simulink model "GLR_recorded_data"  (R2024b)
settings: Solver=VariableStepAuto  StartTime=0.0  StopTime=45  RelTol=1e-3
values from neighbouring files (symbols this model uses):
  G_r1u2_d = c2d(G_r1u2,T_s, 'tustin')    [threeDiskOscillator.m]
  G_r1y1_d = c2d(G_r1y1,T_s, 'tustin')    [threeDiskOscillator.m]
  G_r1y2_d = c2d(G_r1y2,T_s, 'tustin')    [threeDiskOscillator.m]
  G_r1y3_d = c2d(G_r1y3,T_s, 'tustin')    [threeDiskOscillator.m]
  G_r2y2_d = c2d(G_r2y2,T_s, 'tustin')    [threeDiskOscillator.m]
  G_r2y3_d = c2d(G_r2y3,T_s, 'tustin')    [threeDiskOscillator.m]
  h = double(vpasolve(eq_1,gg))    [threeDiskOscillator.m]
  mu_0 = -6.2064e-07    [threeDiskOscillator.m]
  sigma_r2 = 3.6238e-05    [threeDiskOscillator.m]
  T_s = 0.004    [threeDiskOscillator.m]
undefined symbols (not defined in the file or in its folder): M
settings Model: Creator=emma  LastModifiedBy=emma

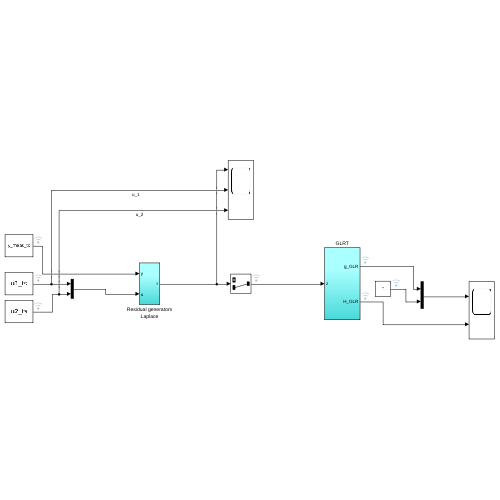
[thumbnail: Simulink's stored preview of the top-level diagram]
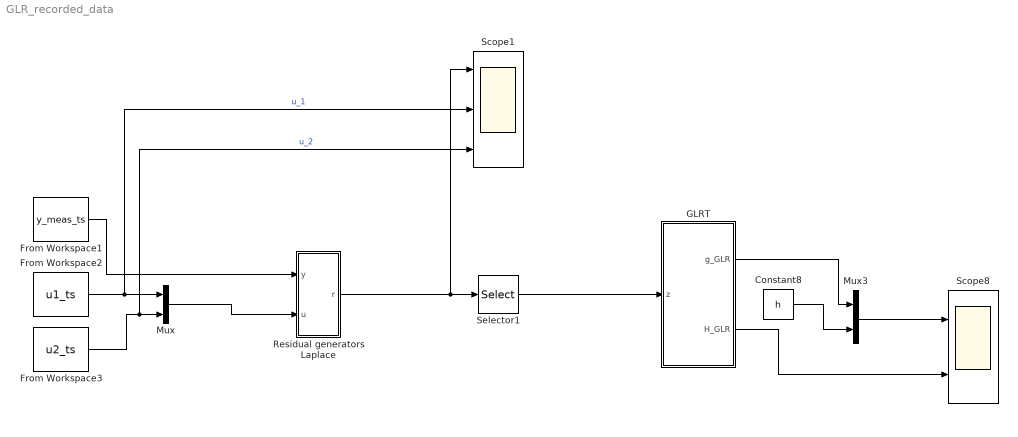
== system GLR_recorded_data ==
  Constant8 : Constant  Value=h
  From Workspace1 : FromWorkspace  VariableName=y_meas_ts  SampleTime=T_s
  From Workspace2 : FromWorkspace  VariableName=u1_ts  SampleTime=T_s
  From Workspace3 : FromWorkspace  VariableName=u2_ts  SampleTime=T_s
  GLRT : Subsystem
  Mux : Mux  Inputs=2
  Mux3 : Mux  Inputs=2
  Residual generators Laplace : Subsystem
  Scope1 : Scope  NumInputPorts=3
  Scope8 : Scope  NumInputPorts=2
  Selector1 : Selector  InputPortWidth=2  IndexOptions=Index vector (dialog)  Indices=[2]  OutputSizes=1
  wires:
  Constant8/1 -> Mux3/2
  Mux3/1 -> Scope8/1
  GLRT/2(H_GLR) -> Scope8/2
  GLRT/1(g_GLR) -> Mux3/1
  From Workspace2/1 -> Scope1/2, Mux/1  "u_1"
  From Workspace3/1 -> Scope1/3, Mux/2  "u_2"
  Mux/1 -> Residual generators Laplace/2(u)
  From Workspace1/1 -> Residual generators Laplace/1(y)
  Residual generators Laplace/1(r) -> Scope1/1, Selector1/1
  Selector1/1 -> GLRT/1(z)

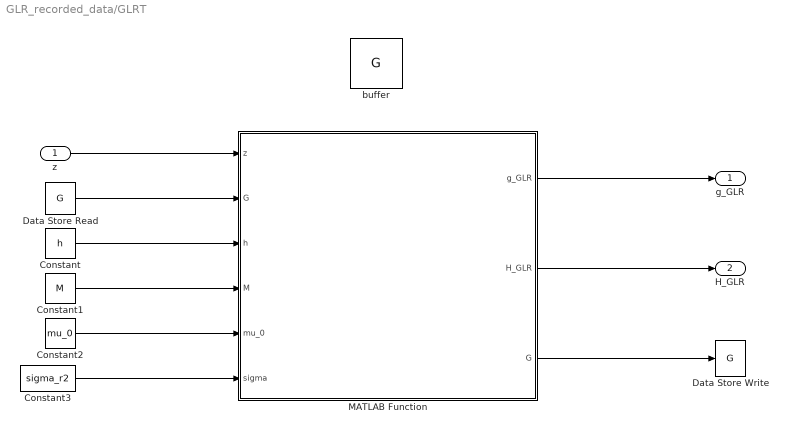
== system GLR_recorded_data/GLRT ==
  z : Inport
  Constant : Constant  Value=h
  Constant1 : Constant  Value=M
  Constant2 : Constant  Value=mu_0
  Constant3 : Constant  Value=sigma_r2
  Data Store Read : DataStoreRead  DataStoreName=G  IndexOptions=Index vector (dialog)  Indices=1  OutputSizes=1
  Data Store Write : DataStoreWrite  DataStoreName=G  IndexOptions=Index vector (dialog)  Indices=1  OutputSizes=1
  MATLAB Function : MATLAB Function  TreatAsAtomicUnit=on
  buffer : DataStoreMemory  DataStoreName=G  WriteAfterWriteMsg=warning  InitialValue=zeros(M,1)  ShowAdditionalParam=off
  g_GLR : Outport  VectorParamsAs1DForOutWhenUnconnected=off
  H_GLR : Outport  Port=2  VectorParamsAs1DForOutWhenUnconnected=off
  wires:
  z/1 -> MATLAB Function/1(z)
  MATLAB Function/1(g_GLR) -> g_GLR/1
  MATLAB Function/2(H_GLR) -> H_GLR/1
  Data Store Read/1 -> MATLAB Function/2("G ")
  MATLAB Function/3(G) -> Data Store Write/1
  Constant/1 -> MATLAB Function/3(h)
  Constant1/1 -> MATLAB Function/4(M)
  Constant2/1 -> MATLAB Function/5(mu_0)
  Constant3/1 -> MATLAB Function/6(sigma)

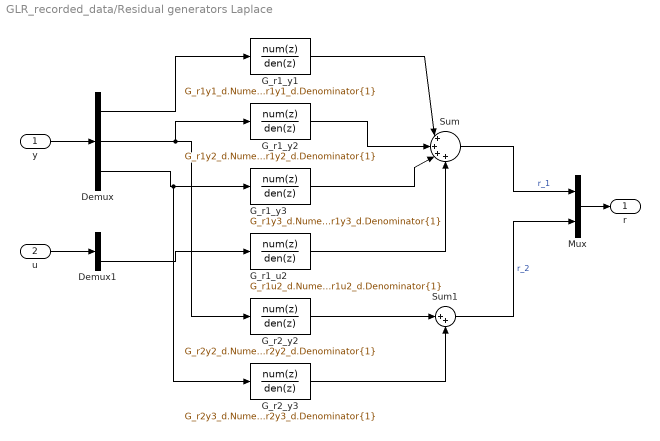
== system GLR_recorded_data/Residual generators Laplace ==
  y : Inport
  u : Inport  Port=2
  Demux : Demux  Outputs=3
  Demux1 : Demux  Outputs=2
  G_r1_u2 : DiscreteTransferFcn  Numerator=G_r1u2_d.Numerator{1}  Denominator=G_r1u2_d.Denominator{1}
  G_r1_y1 : DiscreteTransferFcn  Numerator=G_r1y1_d.Numerator{1}  Denominator=G_r1y1_d.Denominator{1}
  G_r1_y2 : DiscreteTransferFcn  Numerator=G_r1y2_d.Numerator{1}  Denominator=G_r1y2_d.Denominator{1}
  G_r1_y3 : DiscreteTransferFcn  Numerator=G_r1y3_d.Numerator{1}  Denominator=G_r1y3_d.Denominator{1}
  G_r2_y2 : DiscreteTransferFcn  Numerator=G_r2y2_d.Numerator{1}  Denominator=G_r2y2_d.Denominator{1}
  G_r2_y3 : DiscreteTransferFcn  Numerator=G_r2y3_d.Numerator{1}  Denominator=G_r2y3_d.Denominator{1}
  Mux : Mux  Inputs=2
  Sum : Sum  Inputs=|++++
  Sum1 : Sum  Inputs=|++
  r : Outport  VectorParamsAs1DForOutWhenUnconnected=off
  wires:
  y/1 -> Demux/1
  Mux/1 -> r/1
  u/1 -> Demux1/1
  Sum/1 -> Mux/1  "r_1"
  Sum1/1 -> Mux/2  "r_2"
  Demux/1 -> G_r1_y1/1
  G_r1_y1/1 -> Sum/1
  Demux1/2 -> G_r1_u2/1
  G_r2_y2/1 -> Sum1/1
  G_r2_y3/1 -> Sum1/2
  G_r1_y2/1 -> Sum/2
  G_r1_y3/1 -> Sum/3
  G_r1_u2/1 -> Sum/4
  Demux/2 -> G_r2_y2/1, G_r1_y2/1
  Demux/3 -> G_r2_y3/1, G_r1_y3/1

== matlab function GLR_recorded_data/GLRT/MATLAB Function ==
  data: z input; g_GLR output; H_GLR output; G input; G output; h input; M input; mu_0 input; sigma input
function [g_GLR, H_GLR, G] = GLR(z, G, h, M, mu_0, sigma)

G = [G(2:end); z];
maxi = 0;
for i = 1:M
    s = sum(G(M-i+1:end) - mu_0);
    tmp = (s^2) / i;
    if tmp > maxi
        maxi = tmp;
    end
end

g_GLR = maxi/(2*sigma);
H_GLR = (g_GLR>h);
